simulink model "getposition"  (R2019a)
settings: Solver=FixedStepAuto  StartTime=0.0  StopTime=10.0  RelTol=1e-3  EnableMultiTasking=on
libraries: dspstat3 x2
settings Model: Creator=rahelrickenbach  LastModifiedBy=florian
settings SolverCC: PositivePriorityOrder=on
settings OptimizationCC: EnhancedBackFolding=on  PassReuseOutputArgsAs=Individual arguments  MaxStackSize=64  OptimizeBlockOrder=speed  DifferentSizesBufferReuse=on  OptimizationCustomize=off
settings DebuggingCC: ParameterTunabilityLossMsg=error
settings HardwareCC: ProdBitPerPointer=32  ProdBitPerSizeT=32  ProdBitPerPtrDiffT=32  ProdLargestAtomicInteger=Long  ProdLargestAtomicFloat=Double  ProdWordSize=32  ProdLongLongMode=on  ProdHWDeviceType=ARM Compatible->ARM Cortex
settings SFSimCC: MATLABDynamicMemAlloc=off
settings RTWCC: SystemTargetFile=ert.tlc  HardwareBoard=Raspberry Pi  TLCOptions="-aInlineSetEventsForThisBaseRateFcn=TLC_FALSE -aSuppressMultiTaskScheduler=TLC_FALSE  -aRateBasedStepFcn=0"  TemplateMakefile=ert_default_tmf  GenerateReport=on  Toolchain=GNU GCC Raspberry Pi  BuildConfiguration=Faster Runs  IncludeHyperlinkInReport=on  LaunchReport=on  GenerateTraceInfo=on  GenerateTraceReport=on  GenerateTraceReportSl=on  GenerateTraceReportSf=on  GenerateTraceReportEml=on
settings CodeAppCC: ForceParamTrailComments=on  IgnoreCustomStorageClasses=off  OperatorAnnotations=on  SimulinkDataObjDesc=on  SFDataObjDesc=on  InsertBlockDesc=on
settings ERTTargetCC: SupportVariableSizeSignals=on

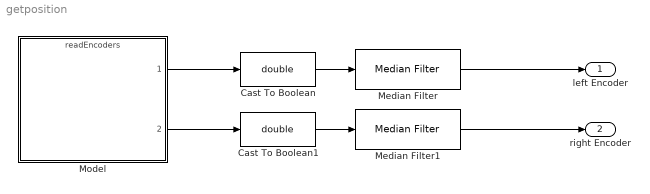
== system getposition ==
  Cast To Boolean : DataTypeConversion  OutDataTypeStr=double
  Cast To Boolean1 : DataTypeConversion  OutDataTypeStr=double
  Median Filter : dspstat3/Median Filter  WindowLength=100  SimulateUsing=Interpreted execution
      settings: SourceProductName=DSP System Toolbox  SourceProductBaseCode=DS
  Median Filter1 : dspstat3/Median Filter  WindowLength=100  SimulateUsing=Interpreted execution
      settings: SourceProductName=DSP System Toolbox  SourceProductBaseCode=DS
  Model : ModelReference  ModelNameDialog=readEncoders.slx  SimulationMode=Normal  ModelReferenceVersion=1.9
  left Encoder : Outport
  "right Encoder " : Outport  Port=2
  wires:
  Median Filter1/1 -> "right Encoder "/1
  Median Filter/1 -> left Encoder/1
  Cast To Boolean1/1 -> Median Filter1/1
  Model/2 -> Cast To Boolean1/1
  Model/1 -> Cast To Boolean/1
  Cast To Boolean/1 -> Median Filter/1
